simulink model "test_chart"  (R2019b)
settings: Solver=VariableStepAuto  StartTime=0.0  StopTime=inf  RelTol=1e-3
settings Model: Creator=nikit  LastModifiedBy=nikit

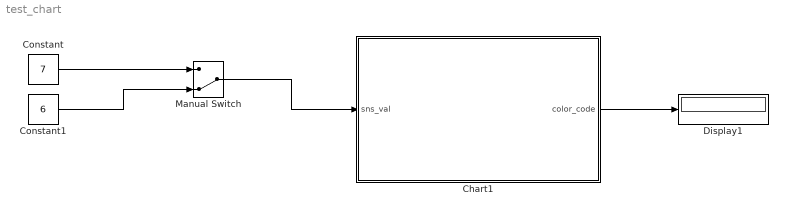
== system test_chart ==
  Chart1 : Stateflow chart  BlockKeywords=__PRM__SERIALIZED__DATA__:Stateflow Chart,Stateflow Diagram  TreatAsAtomicUnit=on
  Constant : Constant  Value=7
  Constant1 : Constant  Value=6
  Display1 : Display
  Manual Switch : ManualSwitch  CurrentSetting=0
  wires:
  Constant1/1 -> Manual Switch/2
  Chart1/1(color_code) -> Display1/1
  Constant/1 -> Manual Switch/1
  Manual Switch/1 -> Chart1/1(sns_val)

== stateflow chart test_chart/Chart1 ==
  state Default
    color_code='red';
  state Check_1
    color_code='green';
  state Check_6
    color_code='blue';
  (default) -> Default
  Default -> Check_1 [order 1] : [sns_val ==1]
  Default -> Check_6 [order 2] : [sns_val ==6]
  Check_1 -> Default [order 2] : [(sns_val ~= 1) & (sns_val ~=6) ]
  Check_6 -> Default [order 2] : [(sns_val ~= 1) & (sns_val ~=6)]
  Check_6 -> Check_1 [order 1] : [sns_val ==1]
  Check_1 -> Check_6 [order 1] : [sns_val==6]
  data: sns_val input; color_code output
